simulink model "LiftControl"  (R2020b)
settings: Solver=VariableStepAuto  StartTime=0.0  StopTime=10.0  RelTol=1e-3
settings Model: Creator=BIDITA PAUL  LastModifiedBy=BIDITA PAUL

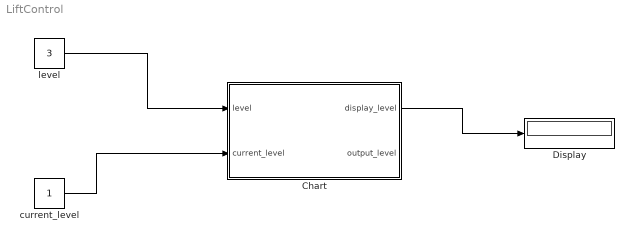
== system LiftControl ==
  Chart : Stateflow chart  TreatAsAtomicUnit=on
  Display : Display
  current_level : Constant
  level : Constant  Value=3
  wires:
  level/1 -> Chart/1(level)
  current_level/1 -> Chart/2(current_level)
  Chart/1(display_level) -> Display/1

== stateflow chart LiftControl/Chart ==
  state REST
    entry:
  state UP
    entry:
    des_level = level;
    output_level = LevelUP(des_level, current_level);
    during:
    exit:
    display_level = current_level;
  state DOWN
    entry:
    des_level = level;
    output_level = LevelDOWN(des_level, current_level);
    during:
    exit:
    display_level = current_level;
  REST -> REST [order 3] : [current_level==level]
  (default) -> REST
  UP -> REST : [level == level_H]
  REST -> UP [order 1] : [level<level_H]
  DOWN -> REST : [level == level_L]
  REST -> DOWN [order 2] : [level>level_L]
  data: des_l function_input; current_l function_output; current_l function_input; des_l function_input; current_l function_output; current_l function_input; level_H local =5; level_L local =0; level input; current_level input; display_level output; des_level local; output_level output
  function current_l = LevelUP(des_l, current_l):
    | function current_l = LevelUP(des_l, current_l)
    | while des_l ~= current_l
    |     current_l = current_l + 1;
    | end
  function current_l = LevelDOWN(des_l, current_l):
    | function current_l = LevelDOWN(des_l, current_l)
    | while des_l ~= current_l
    |     current_l= current_l-1;
    | end
